simulink model "PassStCalib"  (R2024b)
settings: Solver=FixedStepDiscrete  StartTime=0.0  StopTime=10.0  FixedStep=0.01  RelTol=1e-3
model workspace (MAT data in the model file):
  KeSMSwAcsEntryPassStBkReclnUpwdDnwdPosMax_Val : Simulink.Parameter (value not decoded)
  KeSMSwAcsEntryPassStBkReclnUpwdDnwdPosMin_Val : Simulink.Parameter (value not decoded)
  KeSMSwAcsEntryPassStBkReclnUpwdDnwdPos_Val : Simulink.Parameter (value not decoded)
  KeSMSwAcsEntryPassStFrwdBkwdPosMax_Val : Simulink.Parameter (value not decoded)
  KeSMSwAcsEntryPassStFrwdBkwdPosMin_Val : Simulink.Parameter (value not decoded)
  KeSMSwAcsEntryPassStFrwdBkwdPos_Val : Simulink.Parameter (value not decoded)
  KeSMSwAcsMd56PassStBkReclnUpwdDnwdPosMax_Val : Simulink.Parameter (value not decoded)
  KeSMSwAcsMd56PassStBkReclnUpwdDnwdPosMin_Val : Simulink.Parameter (value not decoded)
  KeSMSwAcsMd56PassStBkReclnUpwdDnwdPos_Val : Simulink.Parameter (value not decoded)
  KeSMSwAcsMd56PassStFrwdBkwdPosMax_Val : Simulink.Parameter (value not decoded)
  KeSMSwAcsMd56PassStFrwdBkwdPosMin_Val : Simulink.Parameter (value not decoded)
  KeSMSwAcsMd56PassStFrwdBkwdPos_Val : Simulink.Parameter (value not decoded)
  KeSMSwRevRMDPassStBkReclnUpwdDnwdPosMax_Val : Simulink.Parameter (value not decoded)
  KeSMSwRevRMDPassStBkReclnUpwdDnwdPosMin_Val : Simulink.Parameter (value not decoded)
  KeSMSwRevRMDPassStBkReclnUpwdDnwdPos_Val : Simulink.Parameter (value not decoded)
  KeSMSwRevRMDPassStFrwdBkwdPosMax_Val : Simulink.Parameter (value not decoded)
  KeSMSwRevRMDPassStFrwdBkwdPosMin_Val : Simulink.Parameter (value not decoded)
  KeSMSwRevRMDPassStFrwdBkwdPos_Val : Simulink.Parameter (value not decoded)
symbols that are objects in the model workspace (value not decoded): KeSMSwAcsEntryPassStBkReclnUpwdDnwdPos_Val, KeSMSwAcsEntryPassStBkReclnUpwdDnwdPosMax_Val, KeSMSwAcsEntryPassStBkReclnUpwdDnwdPosMin_Val, KeSMSwAcsEntryPassStFrwdBkwdPos_Val, KeSMSwAcsEntryPassStFrwdBkwdPosMax_Val, KeSMSwAcsEntryPassStFrwdBkwdPosMin_Val, KeSMSwAcsMd56PassStBkReclnUpwdDnwdPos_Val, KeSMSwAcsMd56PassStBkReclnUpwdDnwdPosMax_Val, KeSMSwAcsMd56PassStBkReclnUpwdDnwdPosMin_Val, KeSMSwAcsMd56PassStFrwdBkwdPos_Val, KeSMSwAcsMd56PassStFrwdBkwdPosMax_Val, KeSMSwAcsMd56PassStFrwdBkwdPosMin_Val, KeSMSwRevRMDPassStBkReclnUpwdDnwdPos_Val, KeSMSwRevRMDPassStBkReclnUpwdDnwdPosMax_Val, KeSMSwRevRMDPassStBkReclnUpwdDnwdPosMin_Val, KeSMSwRevRMDPassStFrwdBkwdPos_Val, KeSMSwRevRMDPassStFrwdBkwdPosMax_Val, KeSMSwRevRMDPassStFrwdBkwdPosMin_Val
undefined symbols (not defined in the file or in its folder): KeSMSuSecRwStVIPFtrstRefAngle_Val, KeSMSw6sAcsEntryPassStFtUpwdDnwdPos_Val, KeSMSw6sAcsEntryPassStFtUpwdDnwdPosMiax_Val, KeSMSw6sAcsEntryPassStFtUpwdDnwdPosMin_Val, KeSMSw6sAcsExtPassStFtUpwdDnwdPos_Val, KeSMSw6sAcsExtPassStFtUpwdDnwdPosMax_Val, KeSMSw6sAcsExtPassStFtUpwdDnwdPosMin_Val, KeSMSw6sRecoveryPassStStFtUpwdDnwdPos_Val, KeSMSw6sRecoveryPassStStFtUpwdDnwdPosMax_Val, KeSMSw6sRecoveryPassStStFtUpwdDnwdPosMin_Val, KeSMSw6SVIPMdPassStBkReclnUpwdDnwdPosPos_Val, KeSMSw6SVIPMdPassStBkReclnUpwdDnwdPosPosMax_Val, KeSMSw6SVIPMdPassStBkReclnUpwdDnwdPosPosMin_Val, KeSMSw6SVIPMdPassStFrwdBkwdPos2_Val, KeSMSw6SVIPMdPassStFrwdBkwdPosMax2_Val, KeSMSw6SVIPMdPassStFrwdBkwdPosMin2_Val, KeSMSw6SVIPMdPassStFrwdBkwdPosPos_Val, KeSMSw6SVIPMdPassStFrwdBkwdPosPosMax_Val, KeSMSw6SVIPMdPassStFrwdBkwdPosPosMin_Val, KeSMSwAcsEntryPassStFtUpwdDnwdPos_Val, KeSMSwAcsEntryPassStFtUpwdDnwdPosMiax_Val, KeSMSwAcsEntryPassStFtUpwdDnwdPosMin_Val, KeSMSwAcsExtPassStFtUpwdDnwdPos_Val, KeSMSwAcsExtPassStFtUpwdDnwdPosMax_Val, KeSMSwAcsExtPassStFtUpwdDnwdPosMin_Val, KeSMSwAcsMd30PassStBkReclnUpwdDnwdPos1_Val, KeSMSwAcsMd30PassStBkReclnUpwdDnwdPos1Max_Val, KeSMSwAcsMd30PassStBkReclnUpwdDnwdPos1Min_Val, KeSMSwAcsMd30PassStBkReclnUpwdDnwdPos_Val, KeSMSwAcsMd30PassStBkReclnUpwdDnwdPosMax_Val, KeSMSwAcsMd30PassStBkReclnUpwdDnwdPosMin_Val, KeSMSwAcsMd30PassStFldUpwdDnwdPos1_Val, KeSMSwAcsMd30PassStFldUpwdDnwdPos1Max_Val, KeSMSwAcsMd30PassStFldUpwdDnwdPos1Min_Val, KeSMSwAcsMd30PassStFldUpwdDnwdPos_Val, KeSMSwAcsMd30PassStFldUpwdDnwdPosMax_Val, KeSMSwAcsMd30PassStFldUpwdDnwdPosMin_Val, KeSMSwAcsMd30PassStFrwdBkwdPos1_Val, KeSMSwAcsMd30PassStFrwdBkwdPos1Max_Val, KeSMSwAcsMd30PassStFrwdBkwdPos1Min_Val, KeSMSwAcsMd30PassStFrwdBkwdPos_Val, KeSMSwAcsMd30PassStFrwdBkwdPosMax_Val, KeSMSwAcsMd30PassStFrwdBkwdPosMin_Val, KeSMSwAcsMd31PassStBkReclnUpwdDnwdPos1_Val, KeSMSwAcsMd31PassStBkReclnUpwdDnwdPos1Max_Val, KeSMSwAcsMd31PassStBkReclnUpwdDnwdPos1Min_Val, KeSMSwAcsMd31PassStBkReclnUpwdDnwdPos_Val, KeSMSwAcsMd31PassStBkReclnUpwdDnwdPosMax_Val, KeSMSwAcsMd31PassStBkReclnUpwdDnwdPosMin_Val, KeSMSwAcsMd31PassStFldUpwdDnwdPos_Val, KeSMSwAcsMd31PassStFldUpwdDnwdPosMax_Val, KeSMSwAcsMd31PassStFldUpwdDnwdPosMin_Val, KeSMSwAcsMd31PassStFrwdBkwdPos1_Val, KeSMSwAcsMd31PassStFrwdBkwdPos1Max_Val, KeSMSwAcsMd31PassStFrwdBkwdPos1Min_Val, KeSMSwAcsMd31PassStFrwdBkwdPos_Val, KeSMSwAcsMd31PassStFrwdBkwdPosMax_Val, KeSMSwAcsMd31PassStFrwdBkwdPosMin_Val, KeSMSwAcsMd57PassStBkReclnUpwdDnwdPosPos_Val, KeSMSwAcsMd57PassStBkReclnUpwdDnwdPosPosMax_Val ... (+34)
libraries: TrgtPosSelcLib x20
(part 2 of 3)

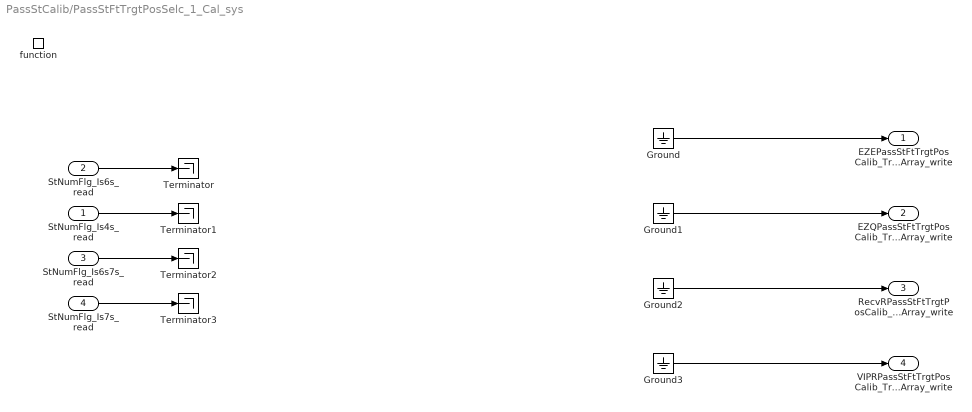
== system PassStCalib/PassStFtTrgtPosSelc_1_Cal_sys ==
  StNumFlg_Is4s_read : Inport
  StNumFlg_Is6s_read : Inport  Port=2
  StNumFlg_Is6s7s_read : Inport  Port=3
  StNumFlg_Is7s_read : Inport  Port=4
  function : TriggerPort  TriggerType=function-call  IsSimulinkFunction=on  FunctionName=PassStFtTrgtPosSelc_1_Cal  VariantControl=(inherit)
  Ground{,1..3} (4 alike) : Ground
  Terminator{,1..3} (4 alike) : Terminator
  EZEPassStFtTrgtPosCalib_TrgtPosArray_write : Outport  VectorParamsAs1DForOutWhenUnconnected=off
      settings: EnsureOutportIsVirtual=on
  EZQPassStFtTrgtPosCalib_TrgtPosArray_write : Outport  Port=2  VectorParamsAs1DForOutWhenUnconnected=off
      settings: EnsureOutportIsVirtual=on
  RecvRPassStFtTrgtPosCalib_TrgtPosArray_write : Outport  Port=3  VectorParamsAs1DForOutWhenUnconnected=off
      settings: EnsureOutportIsVirtual=on
  VIPRPassStFtTrgtPosCalib_TrgtPosArray_write : Outport  Port=4  VectorParamsAs1DForOutWhenUnconnected=off
      settings: EnsureOutportIsVirtual=on
  wires:
  Ground/1 -> EZEPassStFtTrgtPosCalib_TrgtPosArray_write/1
  Ground1/1 -> EZQPassStFtTrgtPosCalib_TrgtPosArray_write/1
  Ground3/1 -> VIPRPassStFtTrgtPosCalib_TrgtPosArray_write/1
  Ground2/1 -> RecvRPassStFtTrgtPosCalib_TrgtPosArray_write/1
  StNumFlg_Is6s_read/1 -> Terminator/1
  StNumFlg_Is4s_read/1 -> Terminator1/1
  StNumFlg_Is6s7s_read/1 -> Terminator2/1
  StNumFlg_Is7s_read/1 -> Terminator3/1

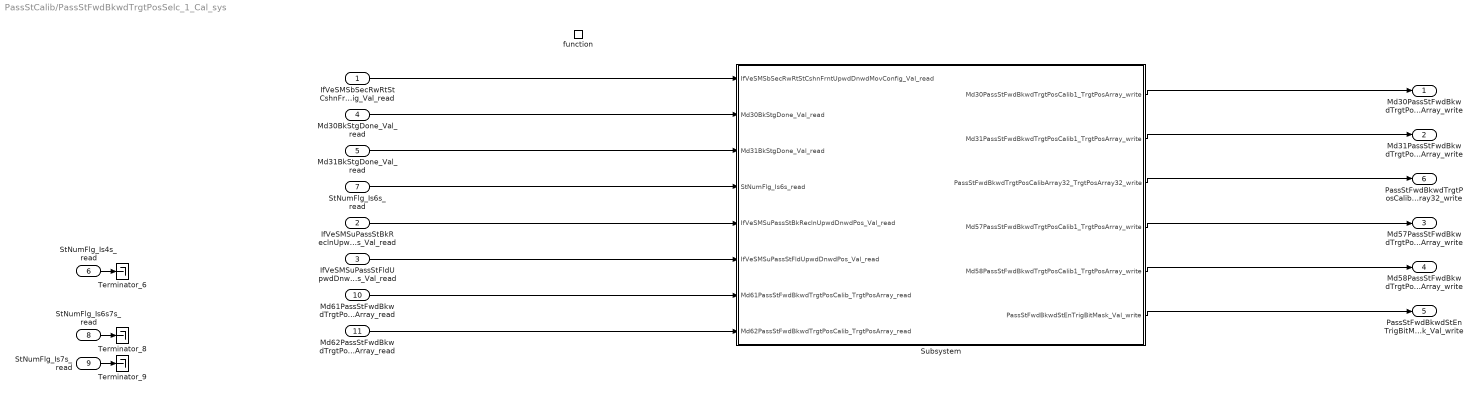
== system PassStCalib/PassStFwdBkwdTrgtPosSelc_1_Cal_sys ==
  IfVeSMSbSecRwRtStCshnFrntUpwdDnwdMovConfig_Val_read : Inport
  IfVeSMSuPassStBkReclnUpwdDnwdPos_Val_read : Inport  Port=2
  IfVeSMSuPassStFldUpwdDnwdPos_Val_read : Inport  Port=3
  Md30BkStgDone_Val_read : Inport  Port=4
  Md31BkStgDone_Val_read : Inport  Port=5
  StNumFlg_Is4s_read : Inport  Port=6
  StNumFlg_Is6s_read : Inport  Port=7
  StNumFlg_Is6s7s_read : Inport  Port=8
  StNumFlg_Is7s_read : Inport  Port=9
  Md61PassStFwdBkwdTrgtPosCalib_TrgtPosArray_read : Inport  Port=10
  Md62PassStFwdBkwdTrgtPosCalib_TrgtPosArray_read : Inport  Port=11
  function : TriggerPort  TriggerType=function-call  IsSimulinkFunction=on  FunctionName=PassStFwdBkwdTrgtPosSelc_1_Cal  VariantControl=(inherit)
  Subsystem : Subsystem
  Terminator_6 : Terminator
  Terminator_8 : Terminator
  Terminator_9 : Terminator
  Md30PassStFwdBkwdTrgtPosCalib1_TrgtPosArray_write : Outport  VectorParamsAs1DForOutWhenUnconnected=off
  Md31PassStFwdBkwdTrgtPosCalib1_TrgtPosArray_write : Outport  Port=2  VectorParamsAs1DForOutWhenUnconnected=off
  Md57PassStFwdBkwdTrgtPosCalib1_TrgtPosArray_write : Outport  Port=3  VectorParamsAs1DForOutWhenUnconnected=off
  Md58PassStFwdBkwdTrgtPosCalib1_TrgtPosArray_write : Outport  Port=4  VectorParamsAs1DForOutWhenUnconnected=off
  PassStFwdBkwdStEnTrigBitMask_Val_write : Outport  Port=5  VectorParamsAs1DForOutWhenUnconnected=off
  PassStFwdBkwdTrgtPosCalibArray32_TrgtPosArray32_write : Outport  Port=6  VectorParamsAs1DForOutWhenUnconnected=off
  wires:
  IfVeSMSbSecRwRtStCshnFrntUpwdDnwdMovConfig_Val_read/1 -> Subsystem/1(IfVeSMSbSecRwRtStCshnFrntUpwdDnwdMovConfig_Val_read)
  IfVeSMSuPassStFldUpwdDnwdPos_Val_read/1 -> Subsystem/6(IfVeSMSuPassStFldUpwdDnwdPos_Val_read)
  Md30BkStgDone_Val_read/1 -> Subsystem/2(Md30BkStgDone_Val_read)
  Md31BkStgDone_Val_read/1 -> Subsystem/3(Md31BkStgDone_Val_read)
  StNumFlg_Is4s_read/1 -> Terminator_6/1
  StNumFlg_Is6s_read/1 -> Subsystem/4(StNumFlg_Is6s_read)
  StNumFlg_Is6s7s_read/1 -> Terminator_8/1
  StNumFlg_Is7s_read/1 -> Terminator_9/1
  Subsystem/1(Md30PassStFwdBkwdTrgtPosCalib1_TrgtPosArray_write) -> Md30PassStFwdBkwdTrgtPosCalib1_TrgtPosArray_write/1
  Subsystem/3(PassStFwdBkwdTrgtPosCalibArray32_TrgtPosArray32_write) -> PassStFwdBkwdTrgtPosCalibArray32_TrgtPosArray32_write/1
  Subsystem/2(Md31PassStFwdBkwdTrgtPosCalib1_TrgtPosArray_write) -> Md31PassStFwdBkwdTrgtPosCalib1_TrgtPosArray_write/1
  Subsystem/4(Md57PassStFwdBkwdTrgtPosCalib1_TrgtPosArray_write) -> Md57PassStFwdBkwdTrgtPosCalib1_TrgtPosArray_write/1
  Subsystem/5(Md58PassStFwdBkwdTrgtPosCalib1_TrgtPosArray_write) -> Md58PassStFwdBkwdTrgtPosCalib1_TrgtPosArray_write/1
  Subsystem/6(PassStFwdBkwdStEnTrigBitMask_Val_write) -> PassStFwdBkwdStEnTrigBitMask_Val_write/1
  IfVeSMSuPassStBkReclnUpwdDnwdPos_Val_read/1 -> Subsystem/5(IfVeSMSuPassStBkReclnUpwdDnwdPos_Val_read)
  Md61PassStFwdBkwdTrgtPosCalib_TrgtPosArray_read/1 -> Subsystem/7(Md61PassStFwdBkwdTrgtPosCalib_TrgtPosArray_read)
  Md62PassStFwdBkwdTrgtPosCalib_TrgtPosArray_read/1 -> Subsystem/8(Md62PassStFwdBkwdTrgtPosCalib_TrgtPosArray_read)

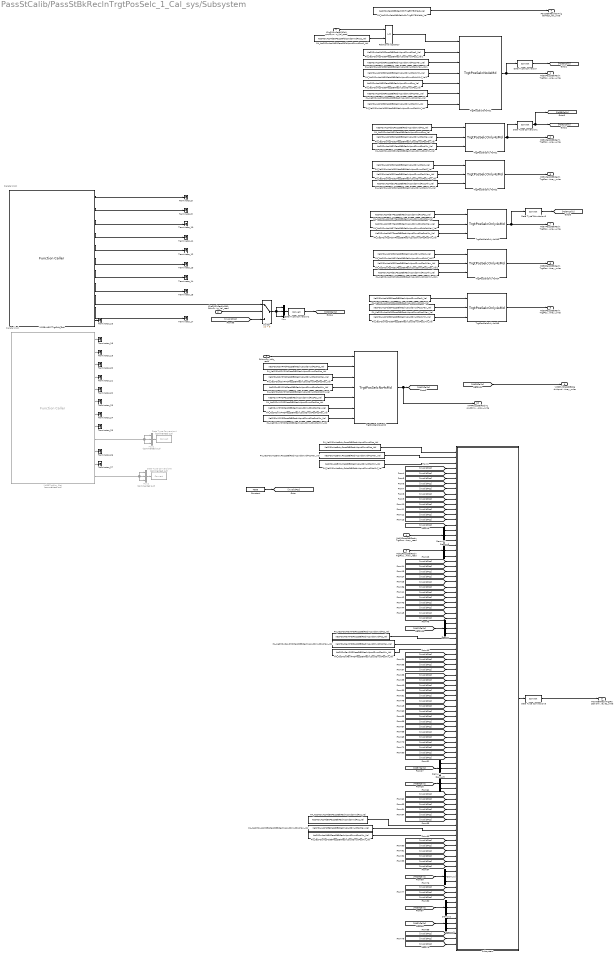
== system PassStCalib/PassStBkReclnTrgtPosSelc_1_Cal_sys/Subsystem ==
  note: Delete block
  note: Delete block
  StNumFlg_Is6s_read : Inport
  IfVeSMSbSecRwRtStCshnFrntUpwdDnwdMovConfig_Val_read : Inport  Port=2
  IfVeSMSuPassStFldUpwdDnwdPos_Val_read : Inport  Port=3
  Md61PassStBkReclnTrgtPosCalib_TrgtPosArray_read : Inport  Port=4
  Md62PassStBkReclnTrgtPosCalib_TrgtPosArray_read : Inport  Port=5
  Constant : Constant  Value=4095  OutDataTypeStr=uint16
  Data Type Conversion{,1..3,5} (5 alike) : DataTypeConversion  SaturateOnIntegerOverflow=off  RndMeth=Floor
  Data Type Conversion4 : DataTypeConversion  Commented=on  SaturateOnIntegerOverflow=off  RndMeth=Floor
  Data Type Conversion6 : DataTypeConversion  Commented=on  SaturateOnIntegerOverflow=off  RndMeth=Floor
  Demux{,1..7} (8 alike) : Demux  Outputs=3
  Md58TrgtPos_Get : FunctionCaller  Commented=on  FunctionPrototype=[SecRwRtStBkReclnTrgtPos,SecRwRtStZeroTrgtPos,SecRwRtStLgrstUpwdDnwdTrgtPos,SecRwRtStLgrstInwdOtwdTrgtPos,ThdRwLtStBkReclnTrgtPos,ThdRwLtStFwdBkwdTrgtPos,ThdRwRtStBkReclnTrgtPos,ThdRwRtStFwdBkwdTrgtPos,PassStBkReclnTrgtPos,PassStFwdBkwdTrgtPos,SecRwRtStFwdBkwdTrgtPos,PassStFldTrgtPos] = Md58TrgtPos_Get()  InputArgumentSpecifications=<Enter example>  OutputArgumentSpecifications=uint16(1), uint16(1), uint16(1), uint16(1), uint16(1), uint16(1), uint16(1), uint16(1), uint16(1), uint16(1), uint16(1), uint16(1)
  Mux : Mux  Inputs=3
  Mux1 : Mux  Commented=on  Inputs=3
  Mux2 : Mux  Commented=on  Inputs=3
  PA_KeSMSw6SVIPMdPassStBkReclnUpwdDnwdPosPosMax_Val : Constant  Value=KeSMSw6SVIPMdPassStBkReclnUpwdDnwdPosPosMax_Val
  PA_KeSMSw6SVIPMdPassStBkReclnUpwdDnwdPosPosMin_Val : Constant  Value=KeSMSw6SVIPMdPassStBkReclnUpwdDnwdPosPosMin_Val
  PA_KeSMSw6SVIPMdPassStBkReclnUpwdDnwdPosPos_Val : Constant  Value=KeSMSw6SVIPMdPassStBkReclnUpwdDnwdPosPos_Val
  PA_KeSMSwAcsEntryPassStBkReclnUpwdDnwdPosMax_Val : Constant  Value=KeSMSwAcsEntryPassStBkReclnUpwdDnwdPosMax_Val
  PA_KeSMSwAcsEntryPassStBkReclnUpwdDnwdPosMin_Val : Constant  Value=KeSMSwAcsEntryPassStBkReclnUpwdDnwdPosMin_Val
  PA_KeSMSwAcsEntryPassStBkReclnUpwdDnwdPos_Val : Constant  Value=KeSMSwAcsEntryPassStBkReclnUpwdDnwdPos_Val
  PA_KeSMSwAcsMd30PassStBkReclnUpwdDnwdPos1Max_Val : Constant  Value=KeSMSwAcsMd30PassStBkReclnUpwdDnwdPos1Max_Val
  PA_KeSMSwAcsMd30PassStBkReclnUpwdDnwdPos1Max_Val1 : Constant  Value=KeSMSwAcsMd30PassStBkReclnUpwdDnwdPos1Max_Val
  PA_KeSMSwAcsMd30PassStBkReclnUpwdDnwdPos1Min_Val : Constant  Value=KeSMSwAcsMd30PassStBkReclnUpwdDnwdPos1Min_Val
  PA_KeSMSwAcsMd30PassStBkReclnUpwdDnwdPos1Min_Val1 : Constant  Value=KeSMSwAcsMd30PassStBkReclnUpwdDnwdPos1Min_Val
  PA_KeSMSwAcsMd30PassStBkReclnUpwdDnwdPos1_Val : Constant  Value=KeSMSwAcsMd30PassStBkReclnUpwdDnwdPos1_Val
  PA_KeSMSwAcsMd30PassStBkReclnUpwdDnwdPos1_Val1 : Constant  Value=KeSMSwAcsMd30PassStBkReclnUpwdDnwdPos1_Val
  PA_KeSMSwAcsMd30PassStBkReclnUpwdDnwdPosMax_Val : Constant  Value=KeSMSwAcsMd30PassStBkReclnUpwdDnwdPosMax_Val
  PA_KeSMSwAcsMd30PassStBkReclnUpwdDnwdPosMin_Val : Constant  Value=KeSMSwAcsMd30PassStBkReclnUpwdDnwdPosMin_Val
  PA_KeSMSwAcsMd30PassStBkReclnUpwdDnwdPos_Val : Constant  Value=KeSMSwAcsMd30PassStBkReclnUpwdDnwdPos_Val
  PA_KeSMSwAcsMd30PassStFldUpwdDnwdPos1_Val : Constant  Value=KeSMSwAcsMd30PassStFldUpwdDnwdPos1_Val
  PA_KeSMSwAcsMd31PassStBkReclnUpwdDnwdPos1Max_Val : Constant  Value=KeSMSwAcsMd31PassStBkReclnUpwdDnwdPos1Max_Val
  PA_KeSMSwAcsMd31PassStBkReclnUpwdDnwdPos1Max_Val1 : Constant  Value=KeSMSwAcsMd31PassStBkReclnUpwdDnwdPos1Max_Val
  PA_KeSMSwAcsMd31PassStBkReclnUpwdDnwdPos1Min_Val : Constant  Value=KeSMSwAcsMd31PassStBkReclnUpwdDnwdPos1Min_Val
  PA_KeSMSwAcsMd31PassStBkReclnUpwdDnwdPos1Min_Val1 : Constant  Value=KeSMSwAcsMd31PassStBkReclnUpwdDnwdPos1Min_Val
  PA_KeSMSwAcsMd31PassStBkReclnUpwdDnwdPos1_Val : Constant  Value=KeSMSwAcsMd31PassStBkReclnUpwdDnwdPos1_Val
  PA_KeSMSwAcsMd31PassStBkReclnUpwdDnwdPos1_Val1 : Constant  Value=KeSMSwAcsMd31PassStBkReclnUpwdDnwdPos1_Val
  PA_KeSMSwAcsMd31PassStBkReclnUpwdDnwdPosMax_Val : Constant  Value=KeSMSwAcsMd31PassStBkReclnUpwdDnwdPosMax_Val
  PA_KeSMSwAcsMd31PassStBkReclnUpwdDnwdPosMin_Val : Constant  Value=KeSMSwAcsMd31PassStBkReclnUpwdDnwdPosMin_Val
  PA_KeSMSwAcsMd31PassStBkReclnUpwdDnwdPos_Val : Constant  Value=KeSMSwAcsMd31PassStBkReclnUpwdDnwdPos_Val
  PA_KeSMSwAcsMd56PassStBkReclnUpwdDnwdPosMax_Val : Constant  Value=KeSMSwAcsMd56PassStBkReclnUpwdDnwdPosMax_Val
  PA_KeSMSwAcsMd56PassStBkReclnUpwdDnwdPosMin_Val : Constant  Value=KeSMSwAcsMd56PassStBkReclnUpwdDnwdPosMin_Val
  PA_KeSMSwAcsMd56PassStBkReclnUpwdDnwdPos_Val : Constant  Value=KeSMSwAcsMd56PassStBkReclnUpwdDnwdPos_Val
  PA_KeSMSwAcsMd57PassStBkReclnUpwdDnwdPosPosMax_Val : Constant  Value=KeSMSwAcsMd57PassStBkReclnUpwdDnwdPosPosMax_Val
  PA_KeSMSwAcsMd57PassStBkReclnUpwdDnwdPosPosMin_Val : Constant  Value=KeSMSwAcsMd57PassStBkReclnUpwdDnwdPosPosMin_Val
  PA_KeSMSwAcsMd57PassStBkReclnUpwdDnwdPosPos_Val : Constant  Value=KeSMSwAcsMd57PassStBkReclnUpwdDnwdPosPos_Val
  PA_KeSMSwPassStBkReclnEnTrig557BitMask_Val : Constant  Value=KeSMSwPassStBkReclnEnTrig557BitMask_Val
  PA_KeSMSwRevRMDPassStBkReclnUpwdDnwdPosMax_Val : Constant  Value=KeSMSwRevRMDPassStBkReclnUpwdDnwdPosMax_Val
  PA_KeSMSwRevRMDPassStBkReclnUpwdDnwdPosMin_Val : Constant  Value=KeSMSwRevRMDPassStBkReclnUpwdDnwdPosMin_Val
  PA_KeSMSwRevRMDPassStBkReclnUpwdDnwdPos_Val : Constant  Value=KeSMSwRevRMDPassStBkReclnUpwdDnwdPos_Val
  PA_KeSMSwVIPMDPassStBkReclnUpwdDnwdPosPosMax_Val : Constant  Value=KeSMSwVIPMDPassStBkReclnUpwdDnwdPosPosMax_Val
  PA_KeSMSwVIPMDPassStBkReclnUpwdDnwdPosPosMin_Val : Constant  Value=KeSMSwVIPMDPassStBkReclnUpwdDnwdPosPosMin_Val
  PA_KeSMSwVIPMDPassStBkReclnUpwdDnwdPosPos_Val : Constant  Value=KeSMSwVIPMDPassStBkReclnUpwdDnwdPosPos_Val
  Relational Operator : RelationalOperator  OutDataTypeStr=boolean  RndMeth=Simplest  InputSameDT=off
  Subsystem : Subsystem
  Switch : Switch  Criteria=u2 > Threshold  SaturateOnIntegerOverflow=off  InputSameDT=off
  Terminator_{8..27} (20 alike) : Terminator
  TrgtPosSelcNo4sMd : TrgtPosSelcLib/TrgtPosSelcNo4sMd  SystemSampleTime=-1  VariantActivationTime=update diagram  AllowFlexibleInterface=on  Latency=0  AutoFrameSizeCalculation=off
  TrgtPosSelcNo4sMd1 : TrgtPosSelcLib/TrgtPosSelcNo4sMd  SystemSampleTime=-1  VariantActivationTime=update diagram  AllowFlexibleInterface=on  Latency=0  AutoFrameSizeCalculation=off
  TrgtPosSelcOnly4sMd{1..5} (5 alike) : TrgtPosSelcLib/TrgtPosSelcOnly4sMd  SystemSampleTime=-1  VariantActivationTime=update diagram  AllowFlexibleInterface=on  Latency=0  AutoFrameSizeCalculation=off
  VIPRExit557TrgtPos_Get : FunctionCaller  FunctionPrototype=[SecRwRtStBkReclnTrgtPos,SecRwRtStZeroTrgtPos,SecRwRtStLgrstUpwdDnwdTrgtPos,SecRwRtStLgrstInwdOtwdTrgtPos,ThdRwLtStBkReclnTrgtPos,ThdRwLtStFwdBkwdTrgtPos,ThdRwRtStBkReclnTrgtPos,ThdRwRtStFwdBkwdTrgtPos,PassStBkReclnTrgtPos,PassStFwdBkwdTrgtPos,SecRwRtStFwdBkwdTrgtPos] = VIPRExit557TrgtPos_Get()  InputArgumentSpecifications=<Enter example>  OutputArgumentSpecifications=uint16(1), uint16(1), uint16(1), uint16(1), uint16(1), uint16(1), uint16(1), uint16(1), uint16(1), uint16(1), uint16(1)
  Md30PassStBkReclnTrgtPosCalib_TrgtPosArray_write : Outport  VectorParamsAs1DForOutWhenUnconnected=off
      settings: EnsureOutportIsVirtual=on
  Md31PassStBkReclnTrgtPosCalib_TrgtPosArray_write : Outport  Port=2  VectorParamsAs1DForOutWhenUnconnected=off
      settings: EnsureOutportIsVirtual=on
  Md31PassStBkReclnTrgtPosCalib1_TrgtPosArray_write : Outport  Port=3  VectorParamsAs1DForOutWhenUnconnected=off
      settings: EnsureOutportIsVirtual=on
  PassStBkReclnEnTrigBitMask_Val_write : Outport  Port=4  VectorParamsAs1DForOutWhenUnconnected=off
      settings: EnsureOutportIsVirtual=on
  PassStBkReclnTrgtPosCalibArray32_TrgtPosArray32_write : Outport  Port=5  VectorParamsAs1DForOutWhenUnconnected=off
      settings: EnsureOutportIsVirtual=on
  VIPRExitPassStBkReclnUpwdDnwdTrgtPosCalib_TrgtPosArray_write : Outport  Port=6  VectorParamsAs1DForOutWhenUnconnected=off
      settings: EnsureOutportIsVirtual=on
  Md57PassStBkReclnTrgtPosCalib_TrgtPosArray_write : Outport  Port=7  VectorParamsAs1DForOutWhenUnconnected=off
      settings: EnsureOutportIsVirtual=on
  Md58PassStBkReclnTrgtPosCalib1_TrgtPosArray_write : Outport  Port=8  VectorParamsAs1DForOutWhenUnconnected=off
      settings: EnsureOutportIsVirtual=on
  Md30PassStBkReclnTrgtPosCalib1_TrgtPosArray_write : Outport  Port=9  VectorParamsAs1DForOutWhenUnconnected=off
      settings: EnsureOutportIsVirtual=on
  VIPRPassStBkReclnUpwdDnwdTrgtPosCalib_TrgtPosArray_write : Outport  Port=10  VectorParamsAs1DForOutWhenUnconnected=off
      settings: EnsureOutportIsVirtual=on
  wires:
  TrgtPosSelcNo4sMd1/1 -> Data Type Conversion/1, Md30PassStBkReclnTrgtPosCalib_TrgtPosArray_write/1
  TrgtPosSelcOnly4sMd1/1 -> Data Type Conversion1/1, Md31PassStBkReclnTrgtPosCalib_TrgtPosArray_write/1
  TrgtPosSelcOnly4sMd2/1 -> Md31PassStBkReclnTrgtPosCalib1_TrgtPosArray_write/1
  PA_KeSMSwAcsMd31PassStBkReclnUpwdDnwdPos1Min_Val/1 -> TrgtPosSelcOnly4sMd2/3
  PA_KeSMSwAcsMd31PassStBkReclnUpwdDnwdPos1Max_Val/1 -> TrgtPosSelcOnly4sMd2/2
  PA_KeSMSwAcsMd31PassStBkReclnUpwdDnwdPos1_Val/1 -> TrgtPosSelcOnly4sMd2/1
  PA_KeSMSwAcsMd31PassStBkReclnUpwdDnwdPosMin_Val/1 -> TrgtPosSelcOnly4sMd1/3
  PA_KeSMSwAcsMd31PassStBkReclnUpwdDnwdPosMax_Val/1 -> TrgtPosSelcOnly4sMd1/2
  PA_KeSMSwAcsMd31PassStBkReclnUpwdDnwdPos_Val/1 -> TrgtPosSelcOnly4sMd1/1
  VIPRExit557TrgtPos_Get/1 -> Terminator_8/1
  VIPRExit557TrgtPos_Get/2 -> Terminator_9/1
  VIPRExit557TrgtPos_Get/3 -> Terminator_10/1
  VIPRExit557TrgtPos_Get/4 -> Terminator_11/1
  VIPRExit557TrgtPos_Get/5 -> Terminator_12/1
  VIPRExit557TrgtPos_Get/6 -> Terminator_13/1
  VIPRExit557TrgtPos_Get/7 -> Terminator_14/1
  VIPRExit557TrgtPos_Get/8 -> Terminator_15/1
  VIPRExit557TrgtPos_Get/10 -> Terminator_17/1
  StNumFlg_Is6s_read/1 -> TrgtPosSelcNo4sMd/1
  PA_KeSMSw6SVIPMdPassStBkReclnUpwdDnwdPosPos_Val/1 -> TrgtPosSelcNo4sMd/2
  PA_KeSMSw6SVIPMdPassStBkReclnUpwdDnwdPosPosMax_Val/1 -> TrgtPosSelcNo4sMd/3
  PA_KeSMSw6SVIPMdPassStBkReclnUpwdDnwdPosPosMin_Val/1 -> TrgtPosSelcNo4sMd/4
  PA_KeSMSwVIPMDPassStBkReclnUpwdDnwdPosPos_Val/1 -> TrgtPosSelcNo4sMd/5
  PA_KeSMSwVIPMDPassStBkReclnUpwdDnwdPosPosMax_Val/1 -> TrgtPosSelcNo4sMd/6
  PA_KeSMSwVIPMDPassStBkReclnUpwdDnwdPosPosMin_Val/1 -> TrgtPosSelcNo4sMd/7
  TrgtPosSelcNo4sMd/1 -> VIPRPassStBkReclnUpwdDnwdTrgtPosCalib_TrgtPosArray_write/1, [Md12Calib]
  PA_KeSMSwPassStBkReclnEnTrig557BitMask_Val/1 -> PassStBkReclnEnTrigBitMask_Val_write/1
  Subsystem/1(CalibArray32) -> Data Type Conversion3/1
  Constant/1 -> [invalidPos]
  PA_KeSMSwAcsEntryPassStBkReclnUpwdDnwdPos_Val/1 -> Subsystem/1(Md1Pos)
  PA_KeSMSwAcsEntryPassStBkReclnUpwdDnwdPosMax_Val/1 -> Subsystem/2(Md1Max)
  PA_KeSMSwAcsEntryPassStBkReclnUpwdDnwdPosMin_Val/1 -> Subsystem/3(Md1Min)
  [invalidPos] -> Subsystem/4(Md2Pos)
  [invalidPos] -> Subsystem/6(Md2PosMin)
  [invalidPos] -> Subsystem/5(Md2PosMax)
  [invalidPos] -> Subsystem/10(Md4Pos)
  [invalidPos] -> Subsystem/12(Md4PosMin)
  [invalidPos] -> Subsystem/11(Md4PosMax)
  [invalidPos] -> Subsystem/7(Md3Pos)
  [invalidPos] -> Subsystem/9(Md3PosMin)
  [invalidPos] -> Subsystem/8(Md3PosMax)
  Demux6/1 -> Subsystem/16(Md6Pos)
  Demux6/3 -> Subsystem/18(Md6PosMin)
  [invalidPos] -> Subsystem/14(Md5PosMax)
  [invalidPos] -> Subsystem/15(Md5PosMin)
  Demux7/3 -> Subsystem/21(Md7PosMin)
  [invalidPos] -> Subsystem/23(Md8PosMax)
  Demux7/1 -> Subsystem/19(Md7Pos)
  Demux6/2 -> Subsystem/17(Md6PosMax)
  [invalidPos] -> Subsystem/22(Md8Pos)
  Demux7/2 -> Subsystem/20(Md7PosMax)
  [invalidPos] -> Subsystem/24(Md8PosMin)
  [invalidPos] -> Subsystem/13(Md5Pos)
  [invalidPos] -> Subsystem/28(Md10Pos)
  [invalidPos] -> Subsystem/30(Md10PosMin)
  [invalidPos] -> Subsystem/26(Md9PosMax)
  [invalidPos] -> Subsystem/29(Md10PosMax)
  [invalidPos] -> Subsystem/25(Md9Pos)
  [invalidPos] -> Subsystem/40(Md14Pos)
  [invalidPos] -> Subsystem/42(Md14PosMin)
  [invalidPos] -> Subsystem/43(Md15Pos)
  [invalidPos] -> Subsystem/41(Md14PosMax)
  [invalidPos] -> Subsystem/31(Md11Pos)
  [invalidPos] -> Subsystem/47(Md16PosMax)
  [invalidPos] -> Subsystem/27(Md9PosMin)
  [invalidPos] -> Subsystem/45(Md15PosMin)
  PA_KeSMSwRevRMDPassStBkReclnUpwdDnwdPos_Val/1 -> Subsystem/37(Md13Pos)
  [invalidPos] -> Subsystem/33(Md11PosMin)
  Demux/2 -> Subsystem/35(Md12PosMax)
  Demux/1 -> Subsystem/34(Md12Pos)
  [invalidPos] -> Subsystem/32(Md11PosMax)
  PA_KeSMSwRevRMDPassStBkReclnUpwdDnwdPosMax_Val/1 -> Subsystem/38(Md13PosMax)
  PA_KeSMSwRevRMDPassStBkReclnUpwdDnwdPosMin_Val/1 -> Subsystem/39(Md13PosMin)
  Demux/3 -> Subsystem/36(Md12PosMin)
  [invalidPos] -> Subsystem/44(Md15PosMax)
  [invalidPos] -> Subsystem/46(Md16Pos)
  [invalidPos] -> Subsystem/48(Md16PosMin)
  [invalidPos] -> Subsystem/51(Md17PosMin)
  [invalidPos] -> Subsystem/53(Md18PosMax)
  [invalidPos] -> Subsystem/54(Md18PosMin)
  [invalidPos] -> Subsystem/52(Md18Pos)
  [invalidPos] -> Subsystem/49(Md17Pos)
  [invalidPos] -> Subsystem/57(Md19PosMin)
  [invalidPos] -> Subsystem/58(Md20Pos)
  [invalidPos] -> Subsystem/60(Md20PosMin)
  [invalidPos] -> Subsystem/72(Md24PosMin)
  [invalidPos] -> Subsystem/71(Md24PosMax)
  [invalidPos] -> Subsystem/69(Md23PosMin)
  [invalidPos] -> Subsystem/70(Md24Pos)
  [invalidPos] -> Subsystem/55(Md19Pos)
  [invalidPos] -> Subsystem/67(Md23Pos)
  Demux4/2 -> Subsystem/65(Md22PosMax)
  Demux4/3 -> Subsystem/66(Md22PosMin)
  [invalidPos] -> Subsystem/68(Md23PosMax)
  Demux5/1 -> Subsystem/61(Md21Pos)
  Demux4/1 -> Subsystem/64(Md22Pos)
  [invalidPos] -> Subsystem/50(Md17PosMax)
  Demux5/2 -> Subsystem/62(Md21PosMax)
  [invalidPos] -> Subsystem/59(Md20PosMax)
  [invalidPos] -> Subsystem/56(Md19PosMax)
  Demux5/3 -> Subsystem/63(Md21PosMin)
  PA_KeSMSwAcsMd56PassStBkReclnUpwdDnwdPosMin_Val/1 -> Subsystem/75(Md25PosMin)
  [invalidPos] -> Subsystem/77(Md26PosMax)
  [invalidPos] -> Subsystem/78(Md26PosMin)
  [invalidPos] -> Subsystem/76(Md26Pos)
  [invalidPos] -> Subsystem/81(Md27PosMin)
  Demux1/1 -> Subsystem/82(Md28Pos)
  Demux1/3 -> Subsystem/84(Md28PosMin)
  [invalidPos] -> Subsystem/96(Md32PosMin)
  [invalidPos] -> Subsystem/95(Md32PosMax)
  [invalidPos] -> Subsystem/94(Md32Pos)
  [invalidPos] -> Subsystem/79(Md27Pos)
  [invalidPos] -> Subsystem/85(Md29Pos)
  PA_KeSMSwAcsMd56PassStBkReclnUpwdDnwdPosMax_Val/1 -> Subsystem/74(Md25PosMax)
  [invalidPos] -> Subsystem/86(Md29PosMax)
  Demux1/2 -> Subsystem/83(Md28PosMax)
  [invalidPos] -> Subsystem/80(Md27PosMax)
  [invalidPos] -> Subsystem/87(Md29PosMin)
  Mux/1 -> Data Type Conversion2/1
  [Md12Calib] -> Demux/1
  [Md28Calib] -> VIPRExitPassStBkReclnUpwdDnwdTrgtPosCalib_TrgtPosArray_write/1
  IfVeSMSbSecRwRtStCshnFrntUpwdDnwdMovConfig_Val_read/1 -> Switch/2
  VIPRExit557TrgtPos_Get/9 -> Switch/1
  [invalidPos] -> Switch/3
  Switch/1 -> Mux/3, Mux/1, Mux/2
  [Md28Calib] -> Demux1/1
  [Md30Calib] -> Demux2/1
  Demux2/2 -> Subsystem/89(Md30PosMax)
  Demux2/3 -> Subsystem/90(Md30PosMin)
  Demux2/1 -> Subsystem/88(Md30Pos)
  Demux3/1 -> Subsystem/91(Md31Pos)
  Demux3/3 -> Subsystem/93(Md31PosMin)
  Demux3/2 -> Subsystem/92(Md31PosMax)
  [Md31Calib] -> Demux3/1
  Data Type Conversion/1 -> [Md30Calib]
  Data Type Conversion1/1 -> [Md58Calib], [Md31Calib]
  Data Type Conversion2/1 -> [Md28Calib]
  Data Type Conversion3/1 -> PassStBkReclnTrgtPosCalibArray32_TrgtPosArray32_write/1
  VIPRExit557TrgtPos_Get/11 -> Terminator_16/1
  TrgtPosSelcOnly4sMd3/1 -> Data Type Conversion5/1, Md57PassStBkReclnTrgtPosCalib_TrgtPosArray_write/1
  TrgtPosSelcOnly4sMd4/1 -> Md58PassStBkReclnTrgtPosCalib1_TrgtPosArray_write/1
  PA_KeSMSwAcsMd57PassStBkReclnUpwdDnwdPosPosMin_Val/1 -> TrgtPosSelcOnly4sMd3/3
  PA_KeSMSwAcsMd57PassStBkReclnUpwdDnwdPosPosMax_Val/1 -> TrgtPosSelcOnly4sMd3/2
  PA_KeSMSwAcsMd57PassStBkReclnUpwdDnwdPosPos_Val/1 -> TrgtPosSelcOnly4sMd3/1
  PA_KeSMSwAcsMd31PassStBkReclnUpwdDnwdPos1_Val1/1 -> TrgtPosSelcOnly4sMd4/1
  PA_KeSMSwAcsMd31PassStBkReclnUpwdDnwdPos1Max_Val1/1 -> TrgtPosSelcOnly4sMd4/2
  PA_KeSMSwAcsMd31PassStBkReclnUpwdDnwdPos1Min_Val1/1 -> TrgtPosSelcOnly4sMd4/3
  Md58TrgtPos_Get/9 -> Mux1/2, Mux1/1, Mux1/3
  Mux1/1 -> Data Type Conversion4/1
  [Md58Calib] -> Demux4/1
  [Md57Calib] -> Demux5/1
  Data Type Conversion5/1 -> [Md57Calib]
  Mux2/1 -> Data Type Conversion6/1
  Md58TrgtPos_Get/12 -> Mux2/2, Mux2/1, Mux2/3
  Md58TrgtPos_Get/1 -> Terminator_18/1
  Md58TrgtPos_Get/2 -> Terminator_19/1
  Md58TrgtPos_Get/3 -> Terminator_20/1
  Md58TrgtPos_Get/4 -> Terminator_21/1
  Md58TrgtPos_Get/5 -> Terminator_22/1
  Md58TrgtPos_Get/6 -> Terminator_23/1
  Md58TrgtPos_Get/7 -> Terminator_24/1
  Md58TrgtPos_Get/8 -> Terminator_25/1
  Md58TrgtPos_Get/10 -> Terminator_26/1
  Md58TrgtPos_Get/11 -> Terminator_27/1
  TrgtPosSelcOnly4sMd5/1 -> Md30PassStBkReclnTrgtPosCalib1_TrgtPosArray_write/1
  PA_KeSMSwAcsMd30PassStBkReclnUpwdDnwdPos1_Val/1 -> TrgtPosSelcOnly4sMd5/1
  PA_KeSMSwAcsMd30PassStBkReclnUpwdDnwdPos1Max_Val/1 -> TrgtPosSelcOnly4sMd5/2
  PA_KeSMSwAcsMd30PassStBkReclnUpwdDnwdPos1Min_Val/1 -> TrgtPosSelcOnly4sMd5/3
  IfVeSMSuPassStFldUpwdDnwdPos_Val_read/1 -> Relational Operator/1
  PA_KeSMSwAcsMd30PassStFldUpwdDnwdPos1_Val/1 -> Relational Operator/2
  Relational Operator/1 -> TrgtPosSelcNo4sMd1/1
  PA_KeSMSwAcsMd30PassStBkReclnUpwdDnwdPosMax_Val/1 -> TrgtPosSelcNo4sMd1/6
  PA_KeSMSwAcsMd30PassStBkReclnUpwdDnwdPosMin_Val/1 -> TrgtPosSelcNo4sMd1/7
  PA_KeSMSwAcsMd30PassStBkReclnUpwdDnwdPos_Val/1 -> TrgtPosSelcNo4sMd1/5
  PA_KeSMSwAcsMd30PassStBkReclnUpwdDnwdPos1Min_Val1/1 -> TrgtPosSelcNo4sMd1/4
  PA_KeSMSwAcsMd30PassStBkReclnUpwdDnwdPos1Max_Val1/1 -> TrgtPosSelcNo4sMd1/3
  PA_KeSMSwAcsMd30PassStBkReclnUpwdDnwdPos1_Val1/1 -> TrgtPosSelcNo4sMd1/2
  Md61PassStBkReclnTrgtPosCalib_TrgtPosArray_read/1 -> Demux6/1
  Md62PassStBkReclnTrgtPosCalib_TrgtPosArray_read/1 -> Demux7/1
  PA_KeSMSwAcsMd56PassStBkReclnUpwdDnwdPos_Val/1 -> Subsystem/73(Md25Pos)

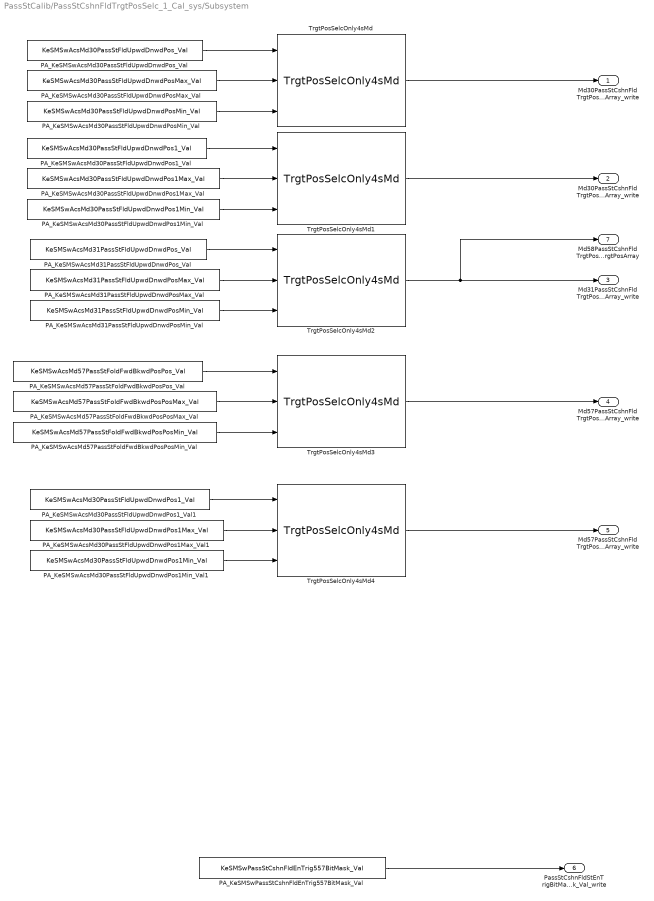
== system PassStCalib/PassStCshnFldTrgtPosSelc_1_Cal_sys/Subsystem ==
  PA_KeSMSwAcsMd30PassStFldUpwdDnwdPos1Max_Val : Constant  Value=KeSMSwAcsMd30PassStFldUpwdDnwdPos1Max_Val
  PA_KeSMSwAcsMd30PassStFldUpwdDnwdPos1Max_Val1 : Constant  Value=KeSMSwAcsMd30PassStFldUpwdDnwdPos1Max_Val
  PA_KeSMSwAcsMd30PassStFldUpwdDnwdPos1Min_Val : Constant  Value=KeSMSwAcsMd30PassStFldUpwdDnwdPos1Min_Val
  PA_KeSMSwAcsMd30PassStFldUpwdDnwdPos1Min_Val1 : Constant  Value=KeSMSwAcsMd30PassStFldUpwdDnwdPos1Min_Val
  PA_KeSMSwAcsMd30PassStFldUpwdDnwdPos1_Val : Constant  Value=KeSMSwAcsMd30PassStFldUpwdDnwdPos1_Val
  PA_KeSMSwAcsMd30PassStFldUpwdDnwdPos1_Val1 : Constant  Value=KeSMSwAcsMd30PassStFldUpwdDnwdPos1_Val
  PA_KeSMSwAcsMd30PassStFldUpwdDnwdPosMax_Val : Constant  Value=KeSMSwAcsMd30PassStFldUpwdDnwdPosMax_Val
  PA_KeSMSwAcsMd30PassStFldUpwdDnwdPosMin_Val : Constant  Value=KeSMSwAcsMd30PassStFldUpwdDnwdPosMin_Val
  PA_KeSMSwAcsMd30PassStFldUpwdDnwdPos_Val : Constant  Value=KeSMSwAcsMd30PassStFldUpwdDnwdPos_Val
  PA_KeSMSwAcsMd31PassStFldUpwdDnwdPosMax_Val : Constant  Value=KeSMSwAcsMd31PassStFldUpwdDnwdPosMax_Val
  PA_KeSMSwAcsMd31PassStFldUpwdDnwdPosMin_Val : Constant  Value=KeSMSwAcsMd31PassStFldUpwdDnwdPosMin_Val
  PA_KeSMSwAcsMd31PassStFldUpwdDnwdPos_Val : Constant  Value=KeSMSwAcsMd31PassStFldUpwdDnwdPos_Val
  PA_KeSMSwAcsMd57PassStFoldFwdBkwdPosPosMax_Val : Constant  Value=KeSMSwAcsMd57PassStFoldFwdBkwdPosPosMax_Val
  PA_KeSMSwAcsMd57PassStFoldFwdBkwdPosPosMin_Val : Constant  Value=KeSMSwAcsMd57PassStFoldFwdBkwdPosPosMin_Val
  PA_KeSMSwAcsMd57PassStFoldFwdBkwdPosPos_Val : Constant  Value=KeSMSwAcsMd57PassStFoldFwdBkwdPosPos_Val
  PA_KeSMSwPassStCshnFldEnTrig557BitMask_Val : Constant  Value=KeSMSwPassStCshnFldEnTrig557BitMask_Val
  TrgtPosSelcOnly4sMd{,1..4} (5 alike) : TrgtPosSelcLib/TrgtPosSelcOnly4sMd  SystemSampleTime=-1  VariantActivationTime=update diagram  AllowFlexibleInterface=on  Latency=0  AutoFrameSizeCalculation=off
  Md30PassStCshnFldTrgtPosCalib_TrgtPosArray_write : Outport  VectorParamsAs1DForOutWhenUnconnected=off
      settings: EnsureOutportIsVirtual=on
  Md30PassStCshnFldTrgtPosCalib1_TrgtPosArray_write : Outport  Port=2  VectorParamsAs1DForOutWhenUnconnected=off
      settings: EnsureOutportIsVirtual=on
  Md31PassStCshnFldTrgtPosCalib_TrgtPosArray_write : Outport  Port=3  VectorParamsAs1DForOutWhenUnconnected=off
      settings: EnsureOutportIsVirtual=on
  Md57PassStCshnFldTrgtPosCalib_TrgtPosArray_write : Outport  Port=4  VectorParamsAs1DForOutWhenUnconnected=off
      settings: EnsureOutportIsVirtual=on
  Md57PassStCshnFldTrgtPosCalib1_TrgtPosArray_write : Outport  Port=5  VectorParamsAs1DForOutWhenUnconnected=off
      settings: EnsureOutportIsVirtual=on
  PassStCshnFldStEnTrigBitMask_Val_write : Outport  Port=6  VectorParamsAs1DForOutWhenUnconnected=off
      settings: EnsureOutportIsVirtual=on
  Md58PassStCshnFldTrgtPosCalib_TrgtPosArray : Outport  Description=|  Port=7  OutDataTypeStr=uint16  PortDimensions=3  VectorParamsAs1DForOutWhenUnconnected=off
      | 0:Pos
      | 1:Max
      | 2:Min
  wires:
  TrgtPosSelcOnly4sMd/1 -> Md30PassStCshnFldTrgtPosCalib_TrgtPosArray_write/1
  TrgtPosSelcOnly4sMd1/1 -> Md30PassStCshnFldTrgtPosCalib1_TrgtPosArray_write/1
  TrgtPosSelcOnly4sMd2/1 -> Md58PassStCshnFldTrgtPosCalib_TrgtPosArray/1, Md31PassStCshnFldTrgtPosCalib_TrgtPosArray_write/1
  PA_KeSMSwAcsMd30PassStFldUpwdDnwdPosMax_Val/1 -> TrgtPosSelcOnly4sMd/2
  PA_KeSMSwAcsMd30PassStFldUpwdDnwdPosMin_Val/1 -> TrgtPosSelcOnly4sMd/3
  PA_KeSMSwAcsMd30PassStFldUpwdDnwdPos_Val/1 -> TrgtPosSelcOnly4sMd/1
  PA_KeSMSwAcsMd30PassStFldUpwdDnwdPos1Max_Val/1 -> TrgtPosSelcOnly4sMd1/2
  PA_KeSMSwAcsMd30PassStFldUpwdDnwdPos1Min_Val/1 -> TrgtPosSelcOnly4sMd1/3
  PA_KeSMSwAcsMd30PassStFldUpwdDnwdPos1_Val/1 -> TrgtPosSelcOnly4sMd1/1
  PA_KeSMSwAcsMd31PassStFldUpwdDnwdPosMax_Val/1 -> TrgtPosSelcOnly4sMd2/2
  PA_KeSMSwAcsMd31PassStFldUpwdDnwdPosMin_Val/1 -> TrgtPosSelcOnly4sMd2/3
  PA_KeSMSwAcsMd31PassStFldUpwdDnwdPos_Val/1 -> TrgtPosSelcOnly4sMd2/1
  PA_KeSMSwAcsMd57PassStFoldFwdBkwdPosPosMax_Val/1 -> TrgtPosSelcOnly4sMd3/2
  PA_KeSMSwAcsMd57PassStFoldFwdBkwdPosPosMin_Val/1 -> TrgtPosSelcOnly4sMd3/3
  PA_KeSMSwAcsMd57PassStFoldFwdBkwdPosPos_Val/1 -> TrgtPosSelcOnly4sMd3/1
  PA_KeSMSwAcsMd30PassStFldUpwdDnwdPos1Min_Val1/1 -> TrgtPosSelcOnly4sMd4/3
  PA_KeSMSwAcsMd30PassStFldUpwdDnwdPos1Max_Val1/1 -> TrgtPosSelcOnly4sMd4/2
  PA_KeSMSwAcsMd30PassStFldUpwdDnwdPos1_Val1/1 -> TrgtPosSelcOnly4sMd4/1
  TrgtPosSelcOnly4sMd3/1 -> Md57PassStCshnFldTrgtPosCalib_TrgtPosArray_write/1
  TrgtPosSelcOnly4sMd4/1 -> Md57PassStCshnFldTrgtPosCalib1_TrgtPosArray_write/1
  PA_KeSMSwPassStCshnFldEnTrig557BitMask_Val/1 -> PassStCshnFldStEnTrigBitMask_Val_write/1
